simulink model "mod_fm"  (R2021a)
settings: Solver=FixedStepAuto  StartTime=0.0  StopTime=15  FixedStep=10e-2  RelTol=1e-3
values from neighbouring files (symbols this model uses):
  fc = fc/1000    (= 4)    [modulacion_fm.m]    (also in modulacion_fm_1.m = 4000; modulacion_fm_voz.m = 100; modulacion_pm_fm.m = 500; modulacion_pm_fm_oct.m = 100)
  kf = 100    [modulacion_pm_fm.m]
  kp = 100    [modulacion_pm_fm.m]    (also in modulacion_pm_fm_oct.m = 15)
settings Model: Creator=Bremdows  LastModifiedBy=Bremdow

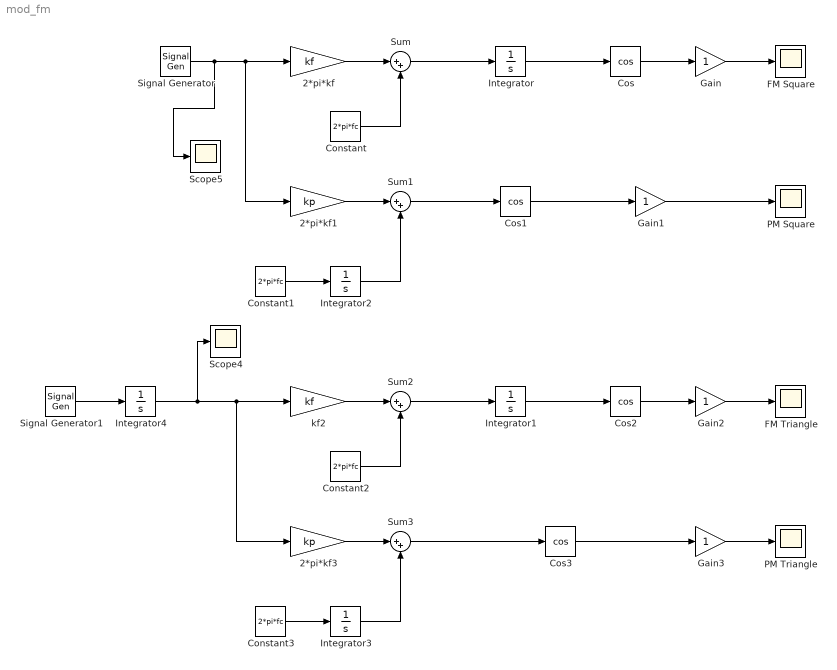
== system mod_fm ==
  2*pi*kf : Gain  Gain=kf
  2*pi*kf1 : Gain  Gain=kp
  2*pi*kf3 : Gain  Gain=kp
  Constant{,1..3} (4 alike) : Constant  Value=2*pi*fc
  Cos{,1..3} (4 alike) : Trigonometry  Operator=cos
  FM Square : Scope
  FM Triangle : Scope
  Gain{,1..3} (4 alike) : Gain
  Integrator{,1..3} (4 alike) : Integrator
  Integrator4 : Integrator  InitialCondition=2
  PM Square : Scope
  PM Triangle : Scope
  Scope4 : Scope
  Scope5 : Scope
  Signal Generator : SignalGenerator  WaveForm=square  Frequency=1.5707  Units=rad/sec
  Signal Generator1 : SignalGenerator  WaveForm=square  Frequency=1.5707  Units=rad/sec
  Sum{,1..3} (4 alike) : Sum  Inputs=|++
  kf2 : Gain  Gain=kf
  wires:
  Cos/1 -> Gain/1
  Integrator/1 -> Cos/1
  Gain/1 -> FM Square/1
  Constant/1 -> Sum/2
  Sum/1 -> Integrator/1
  Signal Generator/1 -> Scope5/1, 2*pi*kf1/1, 2*pi*kf/1
  2*pi*kf/1 -> Sum/1
  Gain1/1 -> PM Square/1
  2*pi*kf1/1 -> Sum1/1
  Sum1/1 -> Cos1/1
  Cos1/1 -> Gain1/1
  Constant1/1 -> Integrator2/1
  Integrator2/1 -> Sum1/2
  Integrator3/1 -> Sum3/2
  Constant3/1 -> Integrator3/1
  Sum3/1 -> Cos3/1
  Gain2/1 -> FM Triangle/1
  kf2/1 -> Sum2/1
  Sum2/1 -> Integrator1/1
  Gain3/1 -> PM Triangle/1
  2*pi*kf3/1 -> Sum3/1
  Cos3/1 -> Gain3/1
  Constant2/1 -> Sum2/2
  Integrator1/1 -> Cos2/1
  Cos2/1 -> Gain2/1
  Signal Generator1/1 -> Integrator4/1
  Integrator4/1 -> Scope4/1, 2*pi*kf3/1, kf2/1
